simulink model "prova"  (R2022b)
settings: Solver=VariableStepAuto  StartTime=0.0  StopTime=.5  RelTol=1e-3
values from neighbouring files (symbols this model uses):
  delta_d_a = 0    [ex2.m]    (also in s270874.mat)
  delta_d_y = 0    [ex2.m]    (also in s270874.mat)
  rho = .25    (= 0.25)    [ex2.m]    (also in s270874.mat)
libraries: cstblocks x2
settings Model: Creator=franc  LastModifiedBy=franc

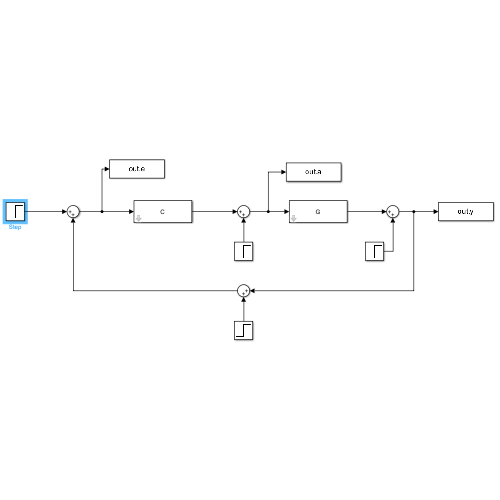
[thumbnail: Simulink's stored preview of the top-level diagram]
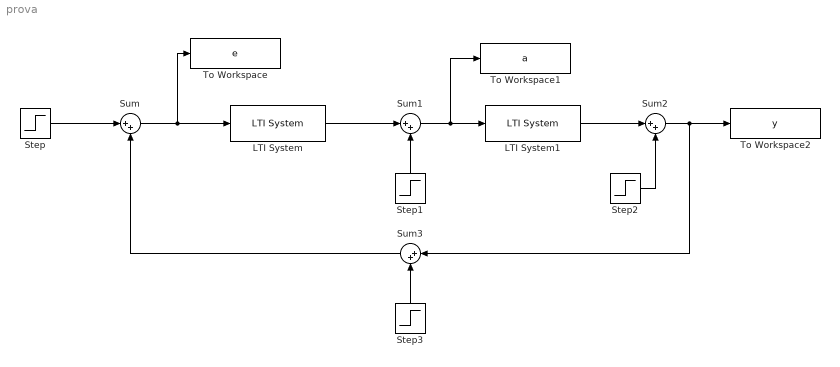
== system prova ==
  LTI System : cstblocks/LTI System  sys=C  IC=[]
  LTI System1 : cstblocks/LTI System  sys=G  IC=[]
  Step : Step  Time=10  After=rho  SampleTime=0
  Step1 : Step  Time=0  After=delta_d_a  SampleTime=0
  Step2 : Step  Time=0  After=delta_d_y  SampleTime=0
  Step3 : Step  Time=0  SampleTime=0
  Sum{,1..3} (4 alike) : Sum  Inputs=|++
  To Workspace : ToWorkspace  VariableName=e  SaveFormat=Timeseries  SampleTime=-1
  To Workspace1 : ToWorkspace  VariableName=a  SaveFormat=Timeseries  SampleTime=-1
  To Workspace2 : ToWorkspace  VariableName=y  SaveFormat=Timeseries  SampleTime=-1
  wires:
  Step/1 -> Sum/1
  Sum/1 -> To Workspace/1, LTI System/1
  LTI System/1 -> Sum1/1
  Step1/1 -> Sum1/2
  LTI System1/1 -> Sum2/1
  Step2/1 -> Sum2/2
  Sum2/1 -> Sum3/1, To Workspace2/1
  Sum3/1 -> Sum/2
  Sum1/1 -> LTI System1/1, To Workspace1/1
  Step3/1 -> Sum3/2
